simulink model "retifier_project"  (R2024b)
settings: Solver=VariableStepAuto  StartTime=0.0  StopTime=0.08  RelTol=1e-3
libraries: spsThyristorLib x4, spsVoltageMeasurementLib x3, spsSeriesRLCBranchLib x2, spsACVoltageSourceLib x1, spsUniversalBridgeLib x1, dspswit3 x1, sps_lib x1
settings Model: Creator=Ahmad  LastModifiedBy=Ahmad

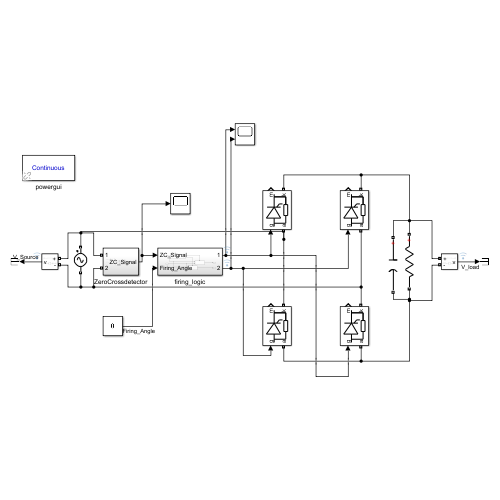
[thumbnail: Simulink's stored preview of the top-level diagram]
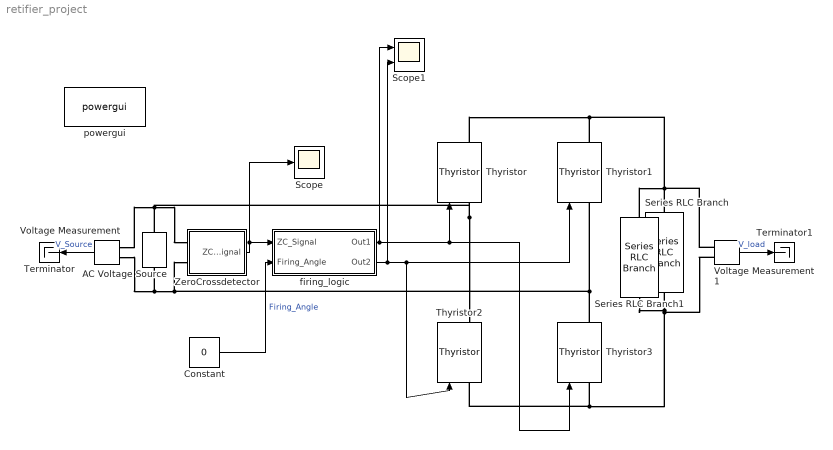
== system retifier_project ==
  AC Voltage Source : spsACVoltageSourceLib/AC Voltage Source  Amplitude=220*sqrt(2)  Phase=0  Frequency=50  SampleTime=0  Measurements=None  BusType=swing  Pref=10e3  Qref=0  Qmin=-inf  Qmax=+inf
  Constant : Constant  Value=0
  Scope : Scope
  Scope1 : Scope  NumInputPorts=2
  Series RLC Branch : spsSeriesRLCBranchLib/Series RLC Branch  LConnTagsString=__new0  RConnTagsString=__new0  BranchType=R  Resistance=1  Inductance=1e-3  SetiL0=off  InitialCurrent=0  Capacitance=1e-6  Setx0=off  InitialVoltage=0  Measurements=None
  Series RLC Branch1 : spsSeriesRLCBranchLib/Series RLC Branch  LConnTagsString=__new0  RConnTagsString=__new0  BranchType=C  Resistance=1  Inductance=1e-3  SetiL0=off  InitialCurrent=0  Capacitance=1  Setx0=off  InitialVoltage=0  Measurements=None
  Terminator : Terminator
  Terminator1 : Terminator
  Thyristor{,1..3} (4 alike) : spsThyristorLib/Thyristor  Ron=0.001  Lon=0  Vf=0.8  IC=0  Rs=500  Cs=250e-9  Measurements=on
  Voltage Measurement : spsVoltageMeasurementLib/Voltage Measurement  PhasorSimulation=off  OutputType=Complex  PSBequivalent=0
  Voltage Measurement1 : spsVoltageMeasurementLib/Voltage Measurement  PhasorSimulation=off  OutputType=Complex  PSBequivalent=0
  ZeroCrossdetector : Subsystem
  firing_logic : Subsystem
  powergui : sps_lib/powergui  Priority=1  SimulationMode=Continuous  SampleTime=50e-6  frequency=60  Iterations=50  frequencyindice=50  Pbase=100e6  ErrMax=1e-4  UnitsV=kV  UnitsW=MW  buscounter=0  FunctionMessages=off  echomessages=off  EnableUseOfTLC=off  CurrentSourceSwitches=off  DisableSnubberDevices=off  DisableRonSwitches=off  DisableVfSwitches=off  DisplayEquations=off  AutomaticDiscreteSolvers=off  SolverType=Tustin/Backward Euler (TBE)  Interpol=off  ExternalGateDelay=off  methode=off  Ts=100  x0status=blocks  SPID=on  SwTol=0  HookPort=off  NonlinearTolerance=1e-4  nMaxIteration=100  ContinueOnMaxIteration=off  RestoreLinks=warning  ResistiveCurrentMeasurement=off  Frange=[0:2:500]  Ylog=off  Xlog=on  ShowGrid=off  save=off  variable=ZData  structure=0  ZoomFFT=off  StartTime=0.0  cycles=1  DisplayStyle=1  fundamental=60  FreqAxis=off  MaxFrequency=1000  frequencyindicesteady=1  RmsSteady=1  display=off
  wires:
  Voltage Measurement/1 -> Terminator/1  "V_Source"
  ZeroCrossdetector/1(ZC_Signal) -> Scope/1, firing_logic/1(ZC_Signal)
  Constant/1 -> firing_logic/2(Firing_Angle)  "Firing_Angle"
  firing_logic/1(Out1) -> Scope1/1, Thyristor3/1, Thyristor/1
  firing_logic/2(Out2) -> Thyristor1/1, Thyristor2/1, Scope1/2
  Voltage Measurement1/1 -> Terminator1/1  "V_load"
  connections:
  Thyristor3/RConn1 -- Voltage Measurement/LConn2 -- AC Voltage Source/LConn1 -- ZeroCrossdetector/LConn2 -- Thyristor1/LConn1
  AC Voltage Source/RConn1 -- Thyristor2/RConn1 -- Thyristor/LConn1 -- ZeroCrossdetector/LConn1 -- Voltage Measurement/LConn1
  Series RLC Branch/LConn1 -- Thyristor1/RConn1 -- Thyristor/RConn1 -- Series RLC Branch1/LConn1 -- Voltage Measurement1/LConn1
  Voltage Measurement1/LConn2 -- Thyristor2/LConn1 -- Thyristor3/LConn1 -- Series RLC Branch1/RConn1 -- Series RLC Branch/RConn1

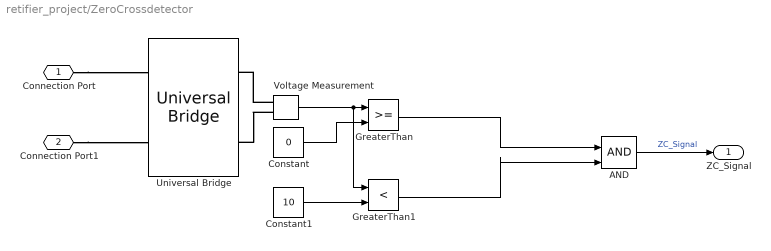
== system retifier_project/ZeroCrossdetector ==
  AND : Logic  IconShape=distinctive  AllPortsSameDT=off  OutDataTypeStr=boolean
  Constant : Constant  Value=0
  Constant1 : Constant  Value=10
  GreaterThan : RelationalOperator  OutDataTypeStr=boolean  RndMeth=Simplest  InputSameDT=off
  GreaterThan1 : RelationalOperator  Operator=<  OutDataTypeStr=boolean  RndMeth=Simplest  InputSameDT=off
  Universal Bridge : spsUniversalBridgeLib/Universal Bridge  Arms=2  SnubberResistance=1e5  SnubberCapacitance=inf  Device=Diodes  Ron=1e-3  Lon=0  ForwardVoltages="[  0  0  ]"  ForwardVoltage=0  GTOparameters=[ 10e-6 , 20e-6 ]  IGBTparameters=[ 1e-6 , 2e-6 ]  Measurements=None  Measurements_2=None  converterType=Rectifier
  Voltage Measurement : spsVoltageMeasurementLib/Voltage Measurement  PhasorSimulation=off  OutputType=Complex  PSBequivalent=0
  Connection Port : PMIOPort  Side=Left
  Connection Port1 : PMIOPort  Port=2  Side=Left
  ZC_Signal : Outport
  wires:
  AND/1 -> ZC_Signal/1  "ZC_Signal"
  Voltage Measurement/1 -> GreaterThan1/1, GreaterThan/1
  Constant/1 -> GreaterThan/2
  GreaterThan/1 -> AND/1
  GreaterThan1/1 -> AND/2
  Constant1/1 -> GreaterThan1/2
  connections:
  Connection Port/RConn1 -- Universal Bridge/LConn1
  Connection Port1/RConn1 -- Universal Bridge/LConn2
  Voltage Measurement/LConn1 -- Universal Bridge/RConn1
  Voltage Measurement/LConn2 -- Universal Bridge/RConn2

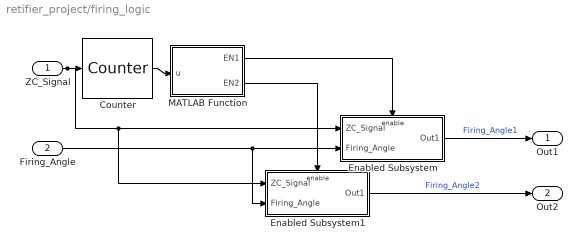
== system retifier_project/firing_logic ==
  ZC_Signal : Inport
  Firing_Angle : Inport  Port=2
  Counter : dspswit3/Counter  Direction=Up  CountEvent=Rising edge  CounterSize=User defined  MaxCount=255  InitialCount=0  Output=Count  HitValue=32  ResetInput=off  SamplesPerFrame=1  Ts=1  CntDtype=double  HitDtype=Logical
  Enabled Subsystem : Subsystem  TreatAsAtomicUnit=on
  Enabled Subsystem1 : Subsystem  TreatAsAtomicUnit=on
  MATLAB Function : MATLAB Function  TreatAsAtomicUnit=on
  Out1 : Outport
  Out2 : Outport  Port=2
  wires:
  ZC_Signal/1 -> Enabled Subsystem1/1(ZC_Signal), Enabled Subsystem/1(ZC_Signal), Counter/1
  Counter/1 -> MATLAB Function/1(u)
  MATLAB Function/1(EN1) -> Enabled Subsystem/Enable
  MATLAB Function/2(EN2) -> Enabled Subsystem1/Enable
  Firing_Angle/1 -> Enabled Subsystem1/2(Firing_Angle), Enabled Subsystem/2(Firing_Angle)
  Enabled Subsystem1/1(Out1) -> Out2/1  "Firing_Angle2"
  Enabled Subsystem/1(Out1) -> Out1/1  "Firing_Angle1"

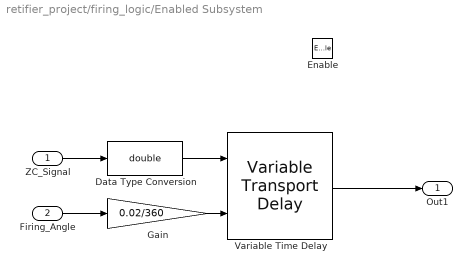
== system retifier_project/firing_logic/Enabled Subsystem ==
  ZC_Signal : Inport
  Firing_Angle : Inport  Port=2
  Enable : EnablePort
  Data Type Conversion : DataTypeConversion  OutDataTypeStr=double  SaturateOnIntegerOverflow=off  RndMeth=Floor
  Gain : Gain  Gain=0.02/360
  Variable Time Delay : VariableTransportDelay  MaximumDelay=10
  Out1 : Outport
  wires:
  Gain/1 -> Variable Time Delay/2
  Firing_Angle/1 -> Gain/1
  ZC_Signal/1 -> Data Type Conversion/1
  Data Type Conversion/1 -> Variable Time Delay/1
  Variable Time Delay/1 -> Out1/1

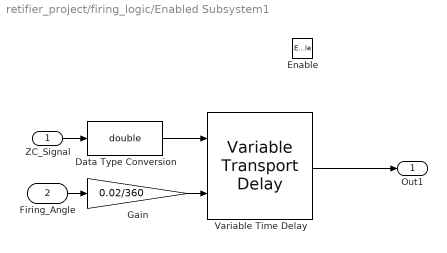
== system retifier_project/firing_logic/Enabled Subsystem1 ==
  ZC_Signal : Inport
  Firing_Angle : Inport  Port=2
  Enable : EnablePort
  Data Type Conversion : DataTypeConversion  OutDataTypeStr=double  SaturateOnIntegerOverflow=off  RndMeth=Floor
  Gain : Gain  Gain=0.02/360
  Variable Time Delay : VariableTransportDelay  MaximumDelay=10
  Out1 : Outport
  wires:
  Data Type Conversion/1 -> Variable Time Delay/1
  Gain/1 -> Variable Time Delay/2
  Variable Time Delay/1 -> Out1/1
  Firing_Angle/1 -> Gain/1
  ZC_Signal/1 -> Data Type Conversion/1

== matlab function retifier_project/firing_logic/MATLAB Function ==
  data: u input; EN1 output; EN2 output
function [EN1,EN2] =fcn(u)

EN1=0;
EN2=0;

if mod(u,2)==0
    EN1=1;
    EN2=0;
end

if mod(u,2)==1
    EN1=0;
    EN2=1;
end
